simulink model "prob_1"  (R2022b)
settings: Solver=VariableStepAuto  StartTime=0.0  StopTime=10.0  RelTol=1e-3
settings Model: Creator=adnzw  LastModifiedBy=adnzw

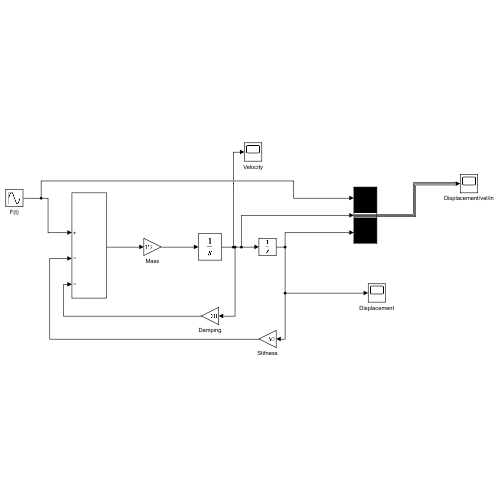
[thumbnail: Simulink's stored preview of the top-level diagram]
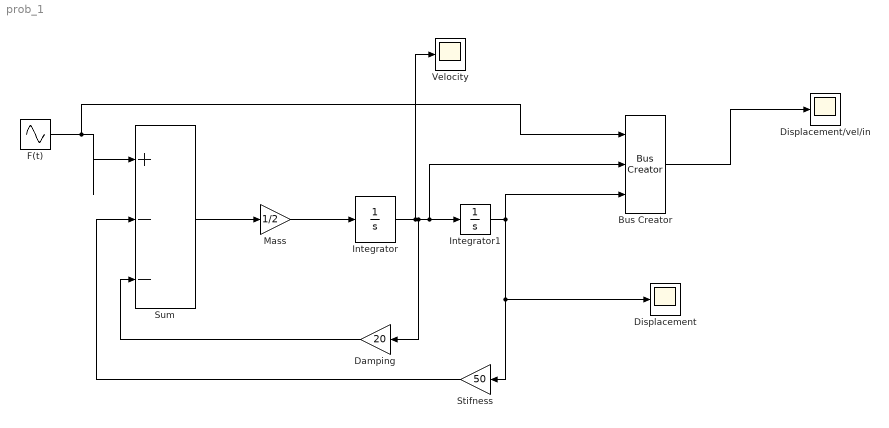
== system prob_1 ==
  Bus Creator : BusCreator  Inputs=3
  Damping : Gain  Gain=20
  Displacement : Scope
  Displacement/vel/in : Scope
  F(t) : Sin  SampleTime=0
  Integrator : Integrator
  Integrator1 : Integrator
  Mass : Gain  Gain=1/2
  Stifness : Gain  Gain=50
  Sum : Sum  Inputs=|+--
  Velocity : Scope
  wires:
  F(t)/1 -> Bus Creator/1, Sum/1
  Sum/1 -> Mass/1
  Mass/1 -> Integrator/1
  Integrator/1 -> Bus Creator/2, Integrator1/1, Damping/1, Velocity/1
  Damping/1 -> Sum/3
  Integrator1/1 -> Stifness/1, Displacement/1, Bus Creator/3
  Stifness/1 -> Sum/2
  Bus Creator/1 -> Displacement/vel/in/1
